simulink model "rctalineal_integrador_bicicleta"  (R2023b)
settings: Solver=VariableStepAuto  StartTime=0.0  StopTime=10.0  RelTol=1e-3
values from neighbouring files (symbols this model uses):
  A = [zeros(2),eye(2);-M_inv * (K0 + (v^2) * K2),-M_inv * (v * C1)]    [Comparacion_Controladores.m]    (also in Realimentacion_Estados_LQR.m)
  B = [zeros(2);M_inv*[1;0],M_inv*[0;1]]    [Comparacion_Controladores.m]    (also in Realimentacion_Estados_LQR.m)
  ke = Kalqr(1:2)    [Comparacion_Controladores.m]
  ki = Kalqr(3)    [Comparacion_Controladores.m]
  x0 = [0.087 ,0.34 ,0.5, 0.5]    [Comparacion_Controladores.m]    (also in Realimentacion_Estados_LQR.m)
settings Model: Creator=paulr  LastModifiedBy=paulr

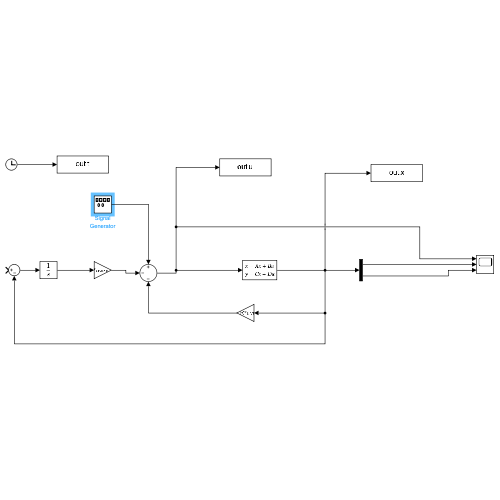
[thumbnail: Simulink's stored preview of the top-level diagram]
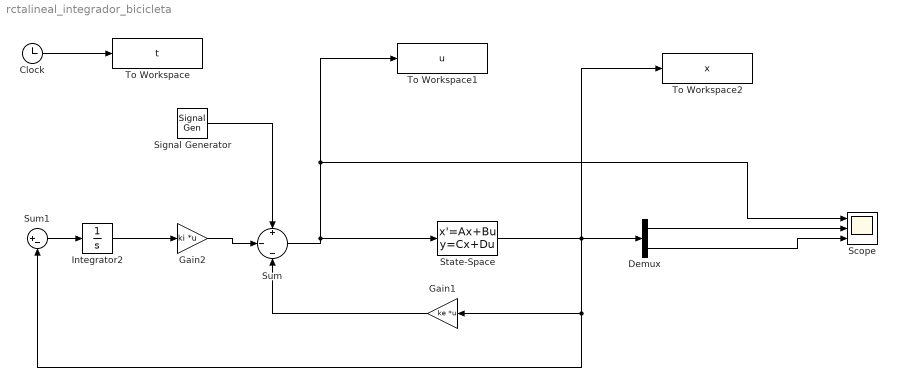
== system rctalineal_integrador_bicicleta ==
  Clock : Clock
  Demux : Demux  Outputs=2
  Gain1 : Gain  Gain=ke  Multiplication=Matrix(K*u) (u vector)
  Gain2 : Gain  Gain=ki  Multiplication=Matrix(K*u) (u vector)
  Integrator2 : Integrator
  Scope : Scope  NumInputPorts=3
  Signal Generator : SignalGenerator  WaveForm=random  Amplitude=0.075  Frequency=2
  State-Space : StateSpace  A=A  B=B  C=eye(4)  D=[0, 0; 0 ,0; 0 ,0; 0 ,0]  InitialCondition=x0
  Sum : Sum  Inputs=+|-|-
  Sum1 : Sum  Inputs=|+-
  To Workspace : ToWorkspace  VariableName=t  SampleTime=-1
  To Workspace1 : ToWorkspace  VariableName=u  SampleTime=-1
  To Workspace2 : ToWorkspace  VariableName=x  SampleTime=-1
  wires:
  State-Space/1 -> To Workspace2/1, Sum1/2, Gain1/1, Demux/1
  Sum/1 -> State-Space/1, To Workspace1/1, Scope/1
  Clock/1 -> To Workspace/1
  Demux/1 -> Scope/2
  Demux/2 -> Scope/3
  Gain1/1 -> Sum/3
  Gain2/1 -> Sum/2
  Integrator2/1 -> Gain2/1
  Sum1/1 -> Integrator2/1
  Signal Generator/1 -> Sum/1
